simulink model "PSFsimu"  (R2017a)
settings: Solver=VariableStepAuto  StartTime=0.0  StopTime=150  RelTol=1e-3
values from neighbouring files (symbols this model uses):
  C_d = minreal(c2d(C, Ts, 'matched'))    [Item3PSF.m]    (also in item3_PSF_comK.m = c2d(C, Ts, 'matched'); psfRapido.m)
  F_d = minreal(c2d(F, Ts, 'matched'))    [Item3PSF.m]    (also in item3_PSF_comK.m = c2d(F, Ts, 'matched'); psfRapido.m)
  Fr = minreal((NumFr/DenFr),1e-2)    [Item3PSF.m]    (also in item3_PSF_comK.m = ((alpha*(z^2) + beta*z + gamma)*(K)*(z^2 - 1.628*z + 0.7312); psfRapido.m = minreal(NumFr/DenFr); robustezPSF.m = minreal(NumFr/DenFr))
  Gq_d = minreal(c2d(Gq, Ts, 'zoh'))    [Item3PSF.m]    (also in item3_PSF_comK.m = c2d(Gq, Ts, 'zoh'); psfRapido.m)
  Gu_d = minreal(c2d(Gu, Ts, 'zoh'))    [Item3PSF.m]    (also in item3_PSF_comK.m = c2d(Gu, Ts, 'zoh'); psfRapido.m)
  Ts = t_5/20    (= 0.075)    [Item3PSF.m]    (also in item3_PSF_comK.m; psfRapido.m; robustezPSF.m)
settings Model: Creator=julia  LastModifiedBy=julia

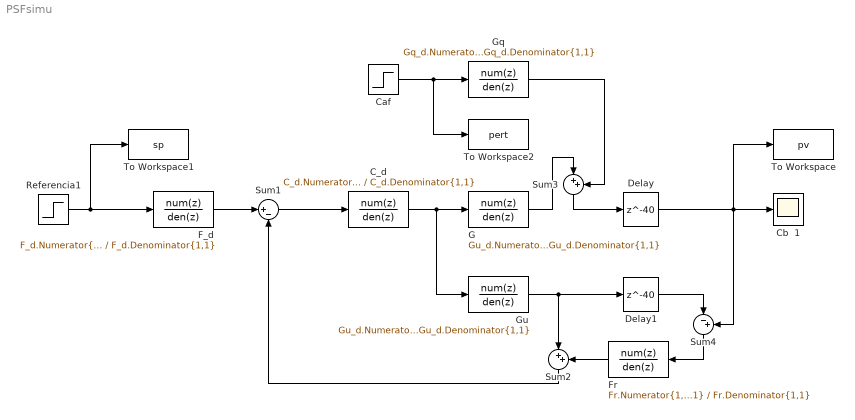
== system PSFsimu ==
  C_d : DiscreteTransferFcn  Numerator=C_d.Numerator{1,1}  Denominator=C_d.Denominator{1,1}  SampleTime=Ts
  Caf : Step  Time=40  After=0.1  SampleTime=0
  Cb  1 : Scope
  Delay : Delay  DelayLength=40  InitialCondition=0
  Delay1 : Delay  DelayLength=40  InitialCondition=0
  F_d : DiscreteTransferFcn  Numerator=F_d.Numerator{1,1}  Denominator=F_d.Denominator{1,1}  SampleTime=Ts
  Fr : DiscreteTransferFcn  Numerator=Fr.Numerator{1,1}  Denominator=Fr.Denominator{1,1}  SampleTime=Ts
  G : DiscreteTransferFcn  Numerator=Gu_d.Numerator{1,1}  Denominator=Gu_d.Denominator{1,1}  SampleTime=Ts
  Gq : DiscreteTransferFcn  Numerator=Gq_d.Numerator{1,1}  Denominator=Gq_d.Denominator{1,1}  SampleTime=Ts
  "Gu " : DiscreteTransferFcn  Numerator=Gu_d.Numerator{1,1}  Denominator=Gu_d.Denominator{1,1}  SampleTime=Ts
  Referencia1 : Step  Time=0  After=0.1  SampleTime=Ts
  Sum1 : Sum  Inputs=|+-
  Sum2 : Sum  Inputs=|++
  Sum3 : Sum  Inputs=|++
  Sum4 : Sum  Inputs=|-+
  To Workspace : ToWorkspace  VariableName=pv  SaveFormat=Timeseries  SampleTime=-1
  To Workspace1 : ToWorkspace  VariableName=sp  SaveFormat=Timeseries  SampleTime=-1
  To Workspace2 : ToWorkspace  VariableName=pert  SaveFormat=Timeseries  SampleTime=-1
  wires:
  Sum1/1 -> C_d/1
  Referencia1/1 -> F_d/1, To Workspace1/1
  Caf/1 -> To Workspace2/1, Gq/1
  F_d/1 -> Sum1/1
  Delay/1 -> To Workspace/1, Sum4/2, Cb  1/1
  C_d/1 -> G/1, "Gu "/1
  "Gu "/1 -> Sum2/1, Delay1/1
  G/1 -> Sum3/1
  Sum3/1 -> Delay/1
  Gq/1 -> Sum3/2
  Fr/1 -> Sum2/2
  Sum2/1 -> Sum1/2
  Delay1/1 -> Sum4/1
  Sum4/1 -> Fr/1
